simulink model "power_factor_measurement"  (R2018a)
settings: Solver=ode23tb  StartTime=0.0  StopTime=10  RelTol=1e-3
libraries: powerlib x5, powerlib_meascontrol x2, pePowerMeasurement x1
settings Model: Creator=sajid  LastModifiedBy=sajid

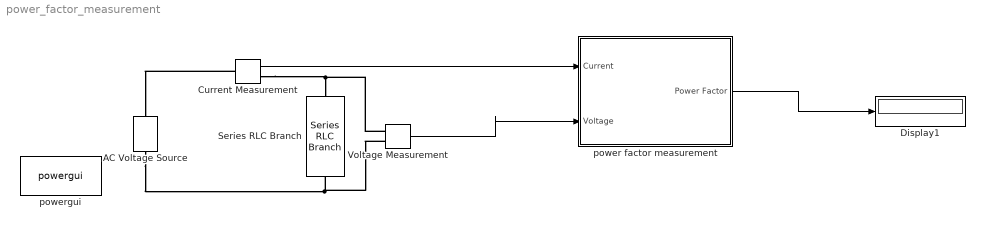
== system power_factor_measurement ==
  AC Voltage Source : powerlib/Electrical Sources/AC Voltage Source  Amplitude=100  Phase=0  Frequency=50  SampleTime=0  Measurements=None  BusType=swing  Pref=10e3  Qref=0  Qmin=-inf  Qmax=+inf
  Current Measurement : powerlib/Measurements/Current Measurement  PhasorSimulation=off  OutputType=Complex  PSBequivalent=0
  Display1 : Display
  Series RLC Branch : powerlib/Elements/Series RLC Branch  LConnTagsString=__new0  RConnTagsString=__new0  BranchType=RL  Resistance=100  Inductance=15  SetiL0=off  InitialCurrent=0  Capacitance=1e-6  Setx0=off  InitialVoltage=0  Measurements=None
  Voltage Measurement : powerlib/Measurements/Voltage Measurement  PhasorSimulation=off  OutputType=Complex  PSBequivalent=0
  "power factor measurement " : Subsystem
      mask help:
      | measures power factor by using formula
      | power factor=Real power divided by apparent power
  powergui : powerlib/powergui  Priority=1  SimulationMode=Continuous  SampleTime=50e-6  frequency=60  Iterations=50  frequencyindice=50  Pbase=100e6  ErrMax=1e-4  UnitsV=kV  UnitsW=MW  buscounter=0  FunctionMessages=off  echomessages=off  EnableUseOfTLC=off  CurrentSourceSwitches=off  DisableSnubberDevices=off  DisableRonSwitches=off  DisableVfSwitches=off  DisplayEquations=off  SolverType=Tustin/Backward Euler (TBE)  Interpol=off  ExternalGateDelay=off  methode=off  Ts=100  x0status=blocks  SPID=on  SwTol=0  HookPort=off  RestoreLinks=warning  ResistiveCurrentMeasurement=off  Frange=[0:2:500]  Ylog=off  Xlog=on  ShowGrid=off  save=off  variable=ZData  structure=0  ZoomFFT=off  StartTime=0.0  cycles=1  DisplayStyle=1  fundamental=60  FreqAxis=off  MaxFrequency=1000  frequencyindicesteady=1  RmsSteady=1  display=off
  wires:
  Current Measurement/1 -> "power factor measurement "/1("Current ")
  Voltage Measurement/1 -> "power factor measurement "/2(Voltage)
  "power factor measurement "/1(Power Factor) -> Display1/1
  connections:
  Current Measurement/LConn1 -- AC Voltage Source/RConn1
  Current Measurement/RConn1 -- Voltage Measurement/LConn1 -- Series RLC Branch/LConn1
  AC Voltage Source/LConn1 -- Voltage Measurement/LConn2 -- Series RLC Branch/RConn1

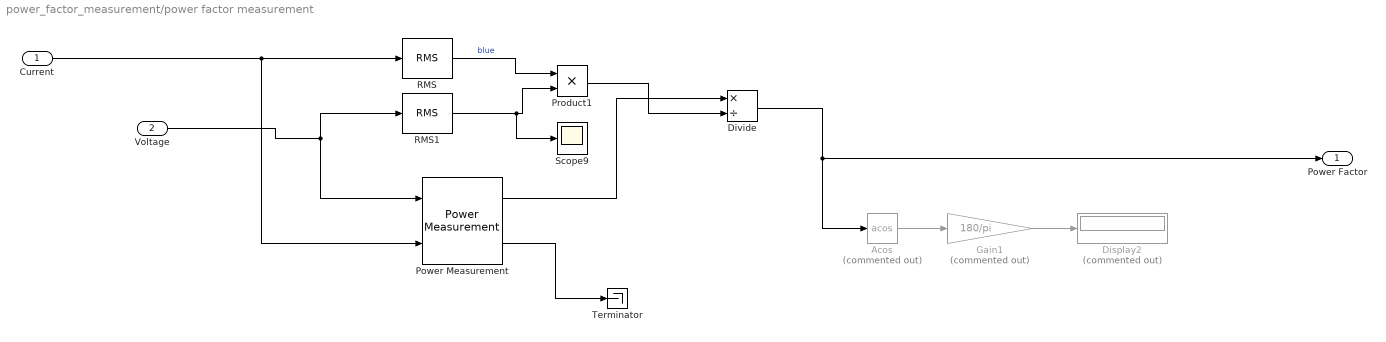
== system power_factor_measurement/power factor measurement  ==
  "Current " : Inport
  Voltage : Inport  Port=2
  Acos : Trigonometry  Commented=on  Operator=acos  OutputSignalType=real
  Display2 : Display  Commented=on
  Divide : Product  Inputs=*/
  Gain1 : Gain  Commented=on  Gain=180/pi
  Power Measurement : pePowerMeasurement/Power Measurement  OverrideUsingVariant=Continuous  F=50  K=[1]  Ts=0
  Product1 : Product
  RMS : powerlib_meascontrol/Measurements/RMS  TrueRMS=on  Freq=60  RMSInit=120  Ts=0
  RMS1 : powerlib_meascontrol/Measurements/RMS  TrueRMS=on  Freq=60  RMSInit=120  Ts=0
  Scope9 : Scope
  Terminator : Terminator
  Power Factor : Outport
  wires:
  Power Measurement/2 -> Terminator/1
  Voltage/1 -> Power Measurement/1, RMS1/1
  Divide/1 -> Power Factor/1, Acos/1
  Gain1/1 -> Display2/1
  Product1/1 -> Divide/2
  "Current "/1 -> Power Measurement/2, RMS/1
  RMS1/1 -> Scope9/1, Product1/2
  Acos/1 -> Gain1/1
  Power Measurement/1 -> Divide/1
  RMS/1 -> Product1/1  "blue"
